simulink model "raw2joint_slx"  (R2016a)
settings: Solver=ode5  StartTime=0.0  StopTime=10.0  FixedStep=0.001  RelTol=1e-3
undefined symbols (not defined in the file or in its folder): Humusoft, MF644
libraries: sldrtlib x4
settings Model: SimulationMode=external  Creator=julianleland  LastModifiedBy=julianleland
settings HardwareCC: ProdBitPerLong=64  ProdLargestAtomicFloat=None  ProdHWDeviceType=Intel->x86-64  TargetBitPerLong=64  TargetBitPerPointer=64  TargetIntDivRoundTo=Zero  TargetEndianess=LittleEndian  TargetWordSize=64  TargetHWDeviceType=Intel->x86-64
settings RTWCC: SystemTargetFile=sldrt.tlc  TemplateMakefile=sldrt.tmf  Description=Simulink Desktop Real-Time  RTWCompilerOptimization=on
settings CodeAppCC: MaxIdLength=95
settings SimulinkDesktopRealTimeCC: TargetPreCompLibLocation=/Applications/MATLAB_R2016a.app/toolbox/sldrt/lib/maci64  TargetLangStandard=C89/C90 (ANSI)  SupportVariableSizeSignals=off

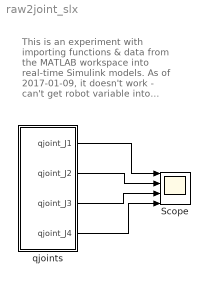
== system raw2joint_slx ==
  note: This is an experiment with importing functions & data from the MATLAB workspace into real-time Simulink models. As of 2017-01-09, it doesn't work - can't get robot variable into Simulink to pass to a Matlab function
  Scope : Scope  NumInputPorts=4
  qjoints : Subsystem
  wires:
  qjoints/1(qjoint_J1) -> Scope/1
  qjoints/2(qjoint_J2) -> Scope/2
  qjoints/3(qjoint_J3) -> Scope/3
  qjoints/4(qjoint_J4) -> Scope/4

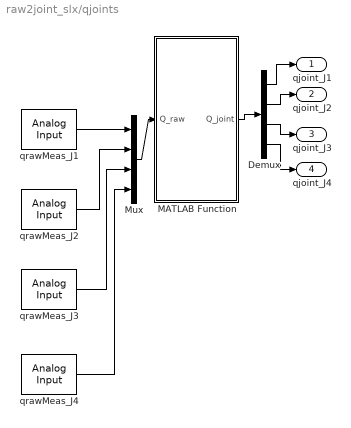
== system raw2joint_slx/qjoints ==
  Demux : Demux
  MATLAB Function : MATLAB Function  TreatAsAtomicUnit=on
  Mux : Mux
  qrawMeas_J1 : sldrtlib/Analog Input  SampleTime=-1  MaxMissedTicks=10  ShowMissedTicks=off  YieldWhenWaiting=off  DrvName=Humusoft/MF644  DrvAddress=4294967295  DrvOptions=585  Channels=1  RangeMode=1  VoltRange=1  DataType=1
      settings: AttributesFormatString=Humusoft\nMF644 [auto]
  qrawMeas_J2 : sldrtlib/Analog Input  SampleTime=-1  MaxMissedTicks=10  ShowMissedTicks=off  YieldWhenWaiting=off  DrvName=Humusoft/MF644  DrvAddress=4294967295  DrvOptions=585  Channels=3  RangeMode=1  VoltRange=1  DataType=1
      settings: AttributesFormatString=Humusoft\nMF644 [auto]
  qrawMeas_J3 : sldrtlib/Analog Input  SampleTime=-1  MaxMissedTicks=10  ShowMissedTicks=off  YieldWhenWaiting=off  DrvName=Humusoft/MF644  DrvAddress=4294967295  DrvOptions=585  Channels=4  RangeMode=1  VoltRange=1  DataType=1
      settings: AttributesFormatString=Humusoft\nMF644 [auto]
  qrawMeas_J4 : sldrtlib/Analog Input  SampleTime=-1  MaxMissedTicks=10  ShowMissedTicks=off  YieldWhenWaiting=off  DrvName=Humusoft/MF644  DrvAddress=4294967295  DrvOptions=585  Channels=5  RangeMode=1  VoltRange=1  DataType=1
      settings: AttributesFormatString=Humusoft\nMF644 [auto]
  qjoint_J1 : Outport
  qjoint_J2 : Outport  Port=2
  qjoint_J3 : Outport  Port=3
  qjoint_J4 : Outport  Port=4
  wires:
  qrawMeas_J4/1 -> Mux/4
  qrawMeas_J3/1 -> Mux/3
  qrawMeas_J2/1 -> Mux/2
  qrawMeas_J1/1 -> Mux/1
  Mux/1 -> MATLAB Function/1(Q_raw)
  MATLAB Function/1(Q_joint) -> Demux/1
  Demux/1 -> qjoint_J1/1
  Demux/2 -> qjoint_J2/1
  Demux/3 -> qjoint_J3/1
  Demux/4 -> qjoint_J4/1

== matlab function raw2joint_slx/qjoints/MATLAB Function ==
  data: Q_joint output; Q_raw input
function Q_joint = raw2joint_slx(Q_raw)
% RAW2JOINT_AT40GW converts raw sensor readings to joint-space positions of
% the AT40GW, where revolute joints 1...3 are in degrees and prismatic
% joint 4 is in mm
% INPUT:
%   robot - robot definition
%   Q_raw - Nx4 matrix of raw joint values (joint 1 is encoder counts, 2..4
%       are in voltages
% OUTPUT:
%   Q_joint - Nx4 matrix of joint-space values in degrees and mm (use
%   deg2rad to convert to radians)

global robot;

Q_joint = zeros(size(Q_raw));

% Joint 1: Encoder counts to degrees
counts2rev = 1/robot.Joint(1).PosSensParams.CountsRev;

Q_joint(:,1) = Q_raw(:,1) .* counts2rev .* 360;

% Joint 2: Voltages to degrees
a = robot.Joint(2).PosSensParams.a_len; % Distance between joint axis and cylinder base axis
b = robot.Joint(2).PosSensParams.b_len; % Distance between joint axis and cylinder attachment point axis
c = robot.Joint(2).PosSensParams.c_len; % Length of cylinder at J_Angle = 0
jointV_Zero = robot.Joint(2).PosSensParams.ZeroVoltage; % Sensor voltage at zero position
jointV_Max = robot.Joint(2).PosLim.Max; % Maximum sensor voltage
jointV_Min = robot.Joint(2).PosLim.Min; % Minimum sensor voltage
sensLen = robot.Joint(2).PosSensParams.SensLen; % Length of joint sensor (allows us to figure out where we are along joint)

% We need to make the orientation of our max/min sensor values match the
% orientation of the joint we're working on.
sensVMax = 10*sign(jointV_Max); 
sensVMin = 10*sign(jointV_Min);
% Find position along sensor of joint zero, relative to center
sensP_Zero = ((jointV_Zero-sensVMin)*((sensLen/2)-(-sensLen/2)))/(sensVMax-sensVMin)+ (-sensLen/2);

% At current voltage, how far away from jointP_Zero are we?
sensP_Cur = ((Q_raw(:,2)-sensVMin)*((sensLen/2)-(-sensLen/2)))/(sensVMax-sensVMin)+ (-sensLen/2);
dSensP = sensP_Zero - sensP_Cur;
J_Len = c - dSensP;

Q_joint(:,2) = (acosd(((J_Len.^2)-(a^2)-(b^2))/(-2*a*b))-acosd(((c^2)-(a^2)-(b^2))/(-2*a*b)));

% Joint 3: Voltages to degrees
a = robot.Joint(3).PosSensParams.a_len; % Distance between joint axis and cylinder base axis
b = robot.Joint(3).PosSensParams.b_len; % Distance between joint axis and cylinder attachment point axis
c = robot.Joint(3).PosSensParams.c_len; % Length of cylinder at J_Angle = 0
jointV_Zero = robot.Joint(3).PosSensParams.ZeroVoltage; % Sensor voltage at zero position
jointV_Max = robot.Joint(3).PosLim.Max; % Maximum sensor voltage
jointV_Min = robot.Joint(3).PosLim.Min; % Minimum sensor voltage
sensLen = robot.Joint(3).PosSensParams.SensLen; % Length of joint sensor (allows us to figure out where we are along joint)

% We need to make the orientation of our max/min sensor values match the
% orientation of the joint we're working on.
sensVMax = 10*sign(jointV_Max); 
sensVMin = 10*sign(jointV_Min);

% Find position along sensor of joint zero, relative to center
sensP_Zero = ((jointV_Zero-sensVMin)*((sensLen/2)-(-sensLen/2)))/(sensVMax-sensVMin)+ (-sensLen/2);

% At current voltage, how far away from jointP_Zero are we?
sensP_Cur = ((Q_raw(:,3)-sensVMin)*((sensLen/2)-(-sensLen/2)))/(sensVMax-sensVMin)+ (-sensLen/2);
dSensP = sensP_Zero - sensP_Cur;
J_Len = c - dSensP;
Q_joint(:,3) = (acosd(((c^2)-(a^2)-(b^2))/(-2*a*b))-acosd(((J_Len.^2)-(a^2)-(b^2))/(-2*a*b)));

% Joint 4: Voltage to mm
a = robot.Joint(4).PosSensParams.a_len; % Distance between joint axis and cylinder base axis
b = robot.Joint(4).PosSensParams.b_len; % Distance between joint axis and cylinder attachment point axis
c = robot.Joint(4).PosSensParams.c_len; % Length of cylinder at J_Angle = 0
jointV_Zero = robot.Joint(4).PosSensParams.ZeroVoltage; % Sensor voltage at zero position
jointV_Max = robot.Joint(4).PosLim.Max; % Maximum sensor voltage
jointV_Min = robot.Joint(4).PosLim.Min; % Minimum sensor voltage
sensLen = robot.Joint(4).PosSensParams.SensLen; % Length of joint sensor (allows us to figure out where we are along joint)

% We need to make the orientation of our max/min sensor values match the
% orientation of the joint we're working on.
sensVMax = 10*sign(jointV_Max); 
sensVMin = 10*sign(jointV_Min);

% Find position along sensor of joint zero, relative to center
sensP_Zero = ((jointV_Zero-sensVMin)*((sensLen/2)-(-sensLen/2)))/(sensVMax-sensVMin)+ (-sensLen/2);

% At current voltage, how far away from jointP_Zero are we?
sensP_Cur = ((Q_raw(:,4)-sensVMin)*((sensLen/2)-(-sensLen/2)))/(sensVMax-sensVMin)+ (-sensLen/2);
dSensP = sensP_Zero - sensP_Cur;
J_Len = c - dSensP;
Q_joint(:,4) = J_Len;

end
